simulink model "csaps_tire_model"  (R2023b)
settings: Solver=ode45  StartTime=0.0  StopTime=20  MaxStep=.01  RelTol=1e-3  EnableMultiTasking=on
undefined symbols (not defined in the file or in its folder): fnval, Fy_from_sa_fz_ia
settings Model: Creator=bglen  LastModifiedBy=bglen
settings SolverCC: AlgebraicLoopSolver=TrustRegion
settings DataIOCC: LimitDataPoints=on  SaveFormat=Array  SignalLoggingSaveFormat=ModelDataLogs  ReturnWorkspaceOutputs=off  SignalLoggingName=sigsOut
settings OptimizationCC: InitFltsAndDblsToZero=on  LifeSpan=inf
settings DebuggingCC: AlgebraicLoopMsg=none  SaveWithParameterizedLinksMsg=none  UnderspecifiedInitializationDetection=Classic  MergeDetectMultiDrivingBlocksExec=none  SignalResolutionControl=TryResolveAllWithWarning  MultiTaskDSMMsg=warning  MultiTaskCondExecSysMsg=none  FcnCallInpInsideContextMsg=warning  UnconnectedInputMsg=warning  UnconnectedOutputMsg=warning  UnconnectedLineMsg=warning  SFUnexpectedBacktrackingDiag=warning  SFNoUnconditionalDefaultTransitionDiag=warning  SFExecutionAtInitializationDiag=none  ArithmeticOperatorsInVariantConditions=warning
settings HardwareCC: ProdBitPerPointer=32  ProdBitPerSizeT=32  ProdBitPerPtrDiffT=32  ProdLargestAtomicFloat=None  ProdIntDivRoundTo=Undefined  ProdEndianess=Unspecified  ProdWordSize=32  ProdHWDeviceType=32-bit Generic  TargetUnknown=on
settings ModelReferenceCC: PropagateSignalLabelsOutOfModel=off
settings CodeAppCC: StateflowObjectComments=on
settings GRTTargetCC: TargetFcnLib=ansi_tfl_tmw.mat  TargetLangStandard=C89/C90 (ANSI)  CombineOutputUpdateFcns=off  GRTInterface=on
settings ConfigComp: CovMetricSettings=dw  CovSaveCumulativeToWorkspaceVar=on  CovSaveSingleToWorkspaceVar=on

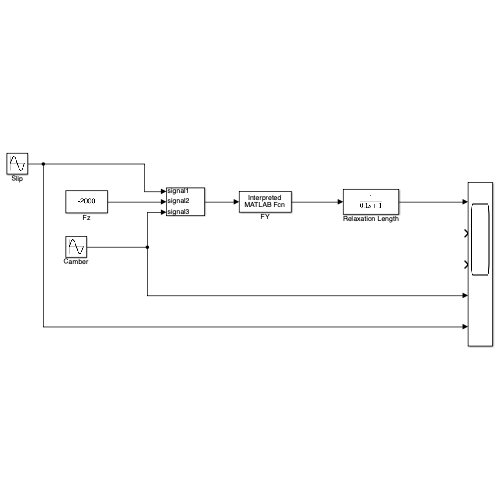
[thumbnail: Simulink's stored preview of the top-level diagram]
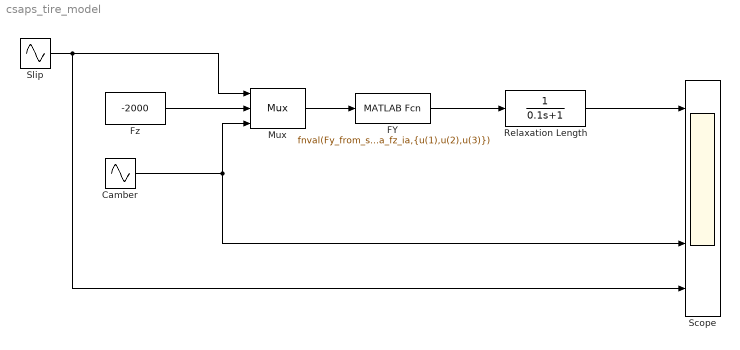
== system csaps_tire_model ==
  Camber : Sin  Amplitude=2  Frequency=40/57.3  SampleTime=0
  FY : MATLABFcn  Tag=Lateral Force  Description=desc  Priority=312271816  MATLABFcn=fnval(Fy_from_sa_fz_ia,{u(1),u(2),u(3)})
  Fz : Constant  Value=-2000
  Mux : Mux  Inputs=3
      settings: DisplayOption=signals
  Relaxation Length : TransferFcn  Denominator=[0.1 1]
  Scope : Scope  NumInputPorts=5
  Slip : Sin  Amplitude=-13  Frequency=70/57.3  SampleTime=0
  wires:
  Mux/1 -> FY/1
  Camber/1 -> Scope/4, Mux/3
  FY/1 -> Relaxation Length/1
  Fz/1 -> Mux/2
  Slip/1 -> Scope/5, Mux/1
  Relaxation Length/1 -> Scope/1
